simulink model "bd_inv_cont_3tank"  (R2021b)
settings: Solver=VariableStepAuto  StartTime=0.0  StopTime=1000  RelTol=1e-3
libraries: dspsrcs4 x4
settings Model: Creator=billtubbs  LastModifiedBy=billtubbs

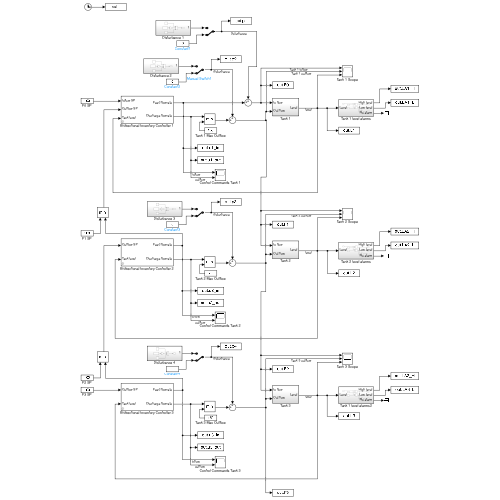
[thumbnail: Simulink's stored preview of the top-level diagram]
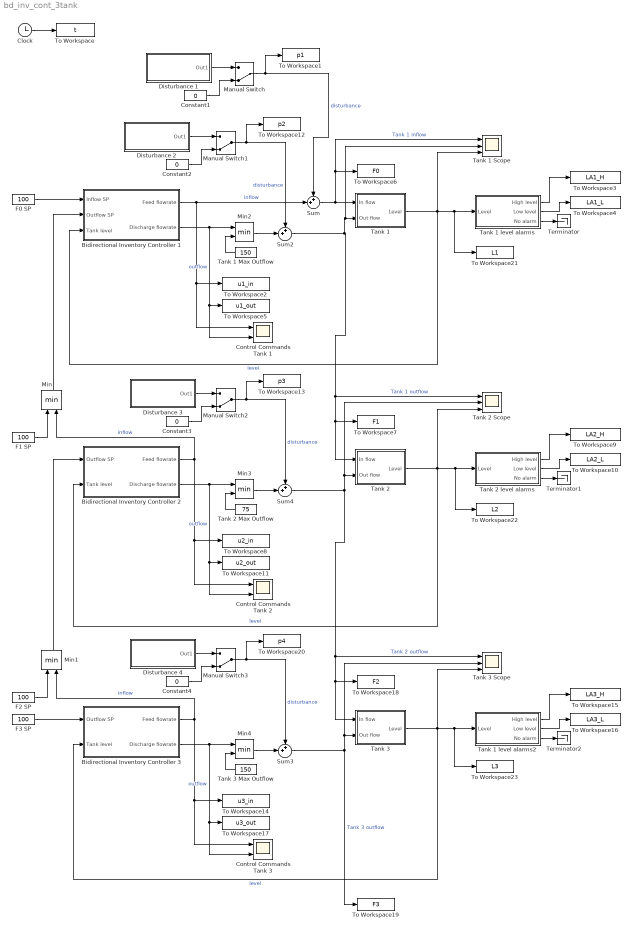
== system bd_inv_cont_3tank ==
  Bidirectional Inventory Controller 1 : Subsystem  mask{K=5, Ti=40, Tsp=40, u_nop=50}
  Bidirectional Inventory Controller 2 : Subsystem  mask{K=5, Ti=40, Tsp=40, u_nop=50}
  Bidirectional Inventory Controller 3 : Subsystem  mask{K=5, Ti=40, Tsp=40, u_nop=50}
  Clock : Clock
  Constant{1..4} (4 alike) : Constant  Value=0  SampleTime=1
  Control Commands Tank 1 : Scope  NumInputPorts=2
  Control Commands Tank 2 : Scope  NumInputPorts=2
  Control Commands Tank 3 : Scope  NumInputPorts=2
  Disturbance 1 : Subsystem
  Disturbance 2 : Subsystem
  Disturbance 3 : Subsystem
  Disturbance 4 : Subsystem
  F0 SP : Constant  Value=100
  F1 SP : Constant  Value=100  VectorParams1D=off
  F2 SP : Constant  Value=100
  F3 SP : Constant  Value=100  VectorParams1D=off
  Manual Switch{,1..3} (4 alike) : ManualSwitch  CurrentSetting=0
  Min{,1..4} (5 alike) : MinMax  Inputs=2
  Sum{,2..4} (4 alike) : Sum  Inputs=++|
  Tank 1 : Subsystem
  Tank 1 Max Outflow : Constant  Value=150
  Tank 1 Scope : Scope  NumInputPorts=3
  Tank 1 level alarms : Subsystem
  Tank 1 level alarms2 : Subsystem
  Tank 2 : Subsystem
  Tank 2 Max Outflow : Constant  Value=75
  Tank 2 Scope : Scope  NumInputPorts=3
  Tank 2 level alarms : Subsystem
  Tank 3 : Subsystem
  Tank 3 Max Outflow : Constant  Value=150
  Tank 3 Scope : Scope  NumInputPorts=3
  Terminator : Terminator
  Terminator1 : Terminator
  Terminator2 : Terminator
  To Workspace : ToWorkspace  VariableName=t  SampleTime=1
  To Workspace1 : ToWorkspace  VariableName=p1  SampleTime=1
      settings: Save2DSignal=2-D array (concatenate along first dimension)
  To Workspace10 : ToWorkspace  VariableName=LA2_L  SampleTime=1
  To Workspace11 : ToWorkspace  VariableName=u2_out  SampleTime=1
  To Workspace12 : ToWorkspace  VariableName=p2  SampleTime=1
      settings: Save2DSignal=2-D array (concatenate along first dimension)
  To Workspace13 : ToWorkspace  VariableName=p3  SampleTime=1
      settings: Save2DSignal=2-D array (concatenate along first dimension)
  To Workspace14 : ToWorkspace  VariableName=u3_in  SampleTime=1
  To Workspace15 : ToWorkspace  VariableName=LA3_H  SampleTime=1
  To Workspace16 : ToWorkspace  VariableName=LA3_L  SampleTime=1
  To Workspace17 : ToWorkspace  VariableName=u3_out  SampleTime=1
  To Workspace18 : ToWorkspace  VariableName=F2  SampleTime=1
  To Workspace19 : ToWorkspace  VariableName=F3  SampleTime=1
  To Workspace2 : ToWorkspace  VariableName=u1_in  SampleTime=1
  To Workspace20 : ToWorkspace  VariableName=p4  SampleTime=1
      settings: Save2DSignal=2-D array (concatenate along first dimension)
  To Workspace21 : ToWorkspace  VariableName=L1  SampleTime=1
  To Workspace22 : ToWorkspace  VariableName=L2  SampleTime=1
  To Workspace23 : ToWorkspace  VariableName=L3  SampleTime=1
  To Workspace3 : ToWorkspace  VariableName=LA1_H  SampleTime=1
  To Workspace4 : ToWorkspace  VariableName=LA1_L  SampleTime=1
  To Workspace5 : ToWorkspace  VariableName=u1_out  SampleTime=1
  To Workspace6 : ToWorkspace  VariableName=F0  SampleTime=1
  To Workspace7 : ToWorkspace  VariableName=F1  SampleTime=1
  To Workspace8 : ToWorkspace  VariableName=u2_in  SampleTime=1
  To Workspace9 : ToWorkspace  VariableName=LA2_H  SampleTime=1
  wires:
  Clock/1 -> To Workspace/1
  Bidirectional Inventory Controller 1/2(Discharge flowrate) -> Min2/1, Control Commands Tank 1/2, To Workspace5/1  "outflow"
  Tank 1 level alarms/3(No alarm) -> Terminator/1
  Sum/1 -> Tank 1/1(In flow), Tank 1 Scope/1, To Workspace6/1  "Tank 1 inflow"
  Manual Switch/1 -> Sum/1, To Workspace1/1  "disturbance"
  Tank 1 level alarms/1(High level) -> To Workspace3/1
  Tank 1 level alarms/2(Low level) -> To Workspace4/1
  Bidirectional Inventory Controller 1/1(Feed flowrate) -> To Workspace2/1, Control Commands Tank 1/1, Sum/2  "inflow"
  Tank 1/1(Level) -> Tank 1 Scope/3, Bidirectional Inventory Controller 1/3(Tank level), To Workspace21/1, Tank 1 level alarms/1(Level)  "level"
  Constant1/1 -> Manual Switch/2
  F0 SP/1 -> Bidirectional Inventory Controller 1/1(Inflow SP)
  F1 SP/1 -> Min/1
  Min1/1 -> Bidirectional Inventory Controller 2/1(Outflow SP)
  Bidirectional Inventory Controller 2/1(Feed flowrate) -> To Workspace8/1, Control Commands Tank 2/1, Min/2  "inflow"
  Tank 2 level alarms/1(High level) -> To Workspace9/1
  Tank 2/1(Level) -> Bidirectional Inventory Controller 2/2(Tank level), Tank 2 Scope/3, To Workspace22/1, Tank 2 level alarms/1(Level)  "level"
  Tank 2 level alarms/2(Low level) -> To Workspace10/1
  Tank 2 level alarms/3(No alarm) -> Terminator1/1
  Sum2/1 -> Tank 2 Scope/1, Tank 2/1(In flow), To Workspace7/1, Tank 1 Scope/2, Tank 1/2(Out flow)  "Tank 1 outflow"
  Bidirectional Inventory Controller 2/2(Discharge flowrate) -> Min3/1, Control Commands Tank 2/2, To Workspace11/1  "outflow"
  F3 SP/1 -> Bidirectional Inventory Controller 3/1(Outflow SP)
  Bidirectional Inventory Controller 3/1(Feed flowrate) -> To Workspace14/1, Control Commands Tank 3/1, Min1/2  "inflow"
  Tank 1 level alarms2/1(High level) -> To Workspace15/1
  Tank 3/1(Level) -> Bidirectional Inventory Controller 3/2(Tank level), Tank 3 Scope/3, To Workspace23/1, Tank 1 level alarms2/1(Level)  "level"
  Tank 1 level alarms2/2(Low level) -> To Workspace16/1
  Tank 1 level alarms2/3(No alarm) -> Terminator2/1
  Bidirectional Inventory Controller 3/2(Discharge flowrate) -> Min4/1, Control Commands Tank 3/2, To Workspace17/1  "outflow"
  Min/1 -> Bidirectional Inventory Controller 1/2(Outflow SP)
  F2 SP/1 -> Min1/1
  Tank 1 Max Outflow/1 -> Min2/2
  Min2/1 -> Sum2/2
  Tank 2 Max Outflow/1 -> Min3/2
  Min3/1 -> Sum4/2
  Sum4/1 -> Tank 3 Scope/1, Tank 3/1(In flow), To Workspace18/1, Tank 2 Scope/2, Tank 2/2(Out flow)  "Tank 2 outflow"
  Min4/1 -> Sum3/2
  Tank 3 Max Outflow/1 -> Min4/2
  Sum3/1 -> To Workspace19/1, Tank 3 Scope/2, Tank 3/2(Out flow)  "Tank 3 outflow"
  Disturbance 1/1(Out1) -> Manual Switch/1
  Constant2/1 -> Manual Switch1/2
  Manual Switch1/1 -> Sum2/1, To Workspace12/1  "disturbance"
  Constant3/1 -> Manual Switch2/2
  Manual Switch2/1 -> Sum4/1, To Workspace13/1  "disturbance"
  Disturbance 3/1(Out1) -> Manual Switch2/1
  Constant4/1 -> Manual Switch3/2
  Disturbance 4/1(Out1) -> Manual Switch3/1
  Manual Switch3/1 -> Sum3/1, To Workspace20/1  "disturbance"
  Disturbance 2/1(Out1) -> Manual Switch1/1

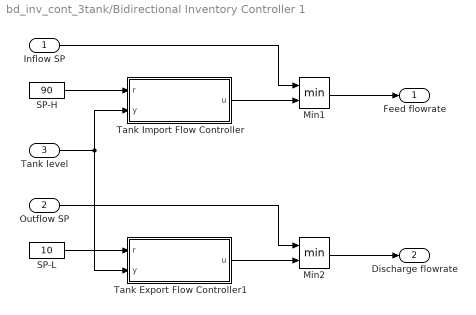
== system bd_inv_cont_3tank/Bidirectional Inventory Controller 1 ==
  Inflow SP : Inport
  Outflow SP : Inport  Port=2
  Tank level : Inport  Port=3
  Min1 : MinMax  Inputs=2
  Min2 : MinMax  Inputs=2
  SP-H : Constant  Value=90
  SP-L : Constant  Value=10
  Tank Export Flow Controller1 : Subsystem
  Tank Import Flow Controller : Subsystem
  Feed flowrate : Outport
  Discharge flowrate : Outport  Port=2
  wires:
  Tank Import Flow Controller/1(u) -> Min1/2
  Outflow SP/1 -> Min2/1
  Tank Export Flow Controller1/1(u) -> Min2/2
  Tank level/1 -> Tank Export Flow Controller1/2(y), Tank Import Flow Controller/2(y)
  SP-H/1 -> Tank Import Flow Controller/1(r)
  SP-L/1 -> Tank Export Flow Controller1/1(r)
  Inflow SP/1 -> Min1/1
  Min1/1 -> Feed flowrate/1
  Min2/1 -> Discharge flowrate/1

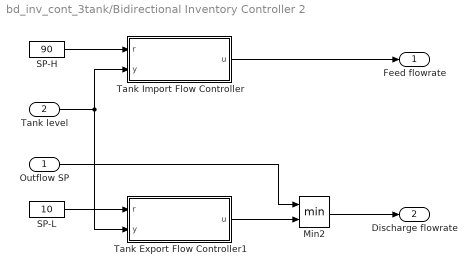
== system bd_inv_cont_3tank/Bidirectional Inventory Controller 2 ==
  Outflow SP : Inport
  Tank level : Inport  Port=2
  Min2 : MinMax  Inputs=2
  SP-H : Constant  Value=90
  SP-L : Constant  Value=10
  Tank Export Flow Controller1 : Subsystem
  Tank Import Flow Controller : Subsystem
  Feed flowrate : Outport
  Discharge flowrate : Outport  Port=2
  wires:
  Tank Import Flow Controller/1(u) -> Feed flowrate/1
  Outflow SP/1 -> Min2/1
  Tank Export Flow Controller1/1(u) -> Min2/2
  Tank level/1 -> Tank Export Flow Controller1/2(y), Tank Import Flow Controller/2(y)
  SP-H/1 -> Tank Import Flow Controller/1(r)
  SP-L/1 -> Tank Export Flow Controller1/1(r)
  Min2/1 -> Discharge flowrate/1

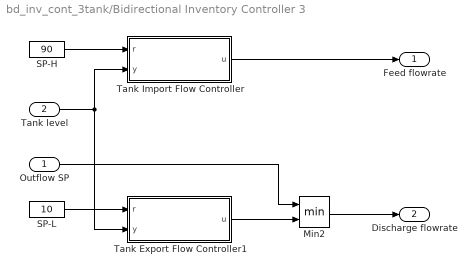
== system bd_inv_cont_3tank/Bidirectional Inventory Controller 3 ==
  Outflow SP : Inport
  Tank level : Inport  Port=2
  Min2 : MinMax  Inputs=2
  SP-H : Constant  Value=90
  SP-L : Constant  Value=10
  Tank Export Flow Controller1 : Subsystem
  Tank Import Flow Controller : Subsystem
  Feed flowrate : Outport
  Discharge flowrate : Outport  Port=2
  wires:
  Tank Import Flow Controller/1(u) -> Feed flowrate/1
  Outflow SP/1 -> Min2/1
  Tank Export Flow Controller1/1(u) -> Min2/2
  Tank level/1 -> Tank Export Flow Controller1/2(y), Tank Import Flow Controller/2(y)
  SP-H/1 -> Tank Import Flow Controller/1(r)
  SP-L/1 -> Tank Export Flow Controller1/1(r)
  Min2/1 -> Discharge flowrate/1

== system bd_inv_cont_3tank/Disturbance 1 ==
  Add : Sum  Inputs=+++
  Colored Noise : dspsrcs4/Colored Noise  Color=pink  InverseFrequencyPower=1  BoundedOutput=off  NumChannels=1  OutputDataType=double  SamplesPerFrame=1  SampleTime=1  RandomStream=mt19937ar with seed  Seed=67  SimulateUsing=Interpreted execution
      settings: SourceProductBaseCode=DS
  Gain : Gain  Gain=3
  Sine Wave : Sin  Amplitude=5  Frequency=1/60  SampleTime=0
  Step : Step  Time=100  After=0  SampleTime=0
  Out1 : Outport
  wires:
  Colored Noise/1 -> Gain/1
  Gain/1 -> Add/2
  Step/1 -> Add/3
  Sine Wave/1 -> Add/1
  Add/1 -> Out1/1

== system bd_inv_cont_3tank/Disturbance 2 ==
  Add : Sum  Inputs=+++
  Colored Noise : dspsrcs4/Colored Noise  Color=pink  InverseFrequencyPower=1  BoundedOutput=off  NumChannels=1  OutputDataType=double  SamplesPerFrame=1  SampleTime=1  RandomStream=mt19937ar with seed  Seed=67  SimulateUsing=Interpreted execution
      settings: SourceProductBaseCode=DS
  Gain : Gain  Gain=3
  Sine Wave : Sin  Amplitude=5  Frequency=1/60  SampleTime=0
  Step : Step  Time=100  After=0  SampleTime=0
  Out1 : Outport
  wires:
  Colored Noise/1 -> Gain/1
  Gain/1 -> Add/2
  Step/1 -> Add/3
  Sine Wave/1 -> Add/1
  Add/1 -> Out1/1

== system bd_inv_cont_3tank/Disturbance 3 ==
  Add : Sum  Inputs=+++
  Colored Noise : dspsrcs4/Colored Noise  Color=pink  InverseFrequencyPower=1  BoundedOutput=off  NumChannels=1  OutputDataType=double  SamplesPerFrame=1  SampleTime=1  RandomStream=mt19937ar with seed  Seed=67  SimulateUsing=Interpreted execution
      settings: SourceProductBaseCode=DS
  Gain : Gain  Gain=3
  Sine Wave : Sin  Amplitude=5  Frequency=1/60  SampleTime=0
  Step : Step  Time=100  After=0  SampleTime=0
  Out1 : Outport
  wires:
  Colored Noise/1 -> Gain/1
  Gain/1 -> Add/2
  Step/1 -> Add/3
  Sine Wave/1 -> Add/1
  Add/1 -> Out1/1

== system bd_inv_cont_3tank/Disturbance 4 ==
  Add : Sum  Inputs=+++
  Colored Noise : dspsrcs4/Colored Noise  Color=pink  InverseFrequencyPower=1  BoundedOutput=off  NumChannels=1  OutputDataType=double  SamplesPerFrame=1  SampleTime=1  RandomStream=mt19937ar with seed  Seed=67  SimulateUsing=Interpreted execution
      settings: SourceProductBaseCode=DS
  Gain : Gain  Gain=3
  Sine Wave : Sin  Amplitude=5  Frequency=1/60  SampleTime=0
  Step : Step  Time=100  After=0  SampleTime=0
  Out1 : Outport
  wires:
  Colored Noise/1 -> Gain/1
  Gain/1 -> Add/2
  Step/1 -> Add/3
  Sine Wave/1 -> Add/1
  Add/1 -> Out1/1

== system bd_inv_cont_3tank/Tank 1 ==
  In flow : Inport
  Out flow : Inport  Port=2
  Gain : Gain  Gain=0.05
  Integrator : Integrator
  Sum : Sum  Inputs=|+-
  Transport Delay : TransportDelay  Commented=on  DelayTime=0
  Level : Outport  InitialOutput=0
  wires:
  Sum/1 -> Gain/1
  Integrator/1 -> Level/1
  In flow/1 -> Sum/1
  Out flow/1 -> Sum/2
  Gain/1 -> Integrator/1

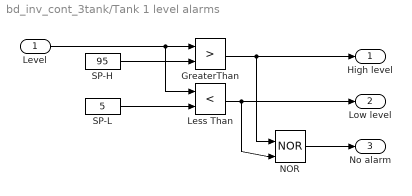
== system bd_inv_cont_3tank/Tank 1 level alarms ==
  Level : Inport
  GreaterThan : RelationalOperator  Operator=>  OutDataTypeStr=boolean  RndMeth=Simplest
  Less Than : RelationalOperator  Operator=<  OutDataTypeStr=boolean  RndMeth=Simplest
  NOR : Logic  Operator=NOR  IconShape=distinctive  AllPortsSameDT=off  OutDataTypeStr=boolean
  SP-H : Constant  Value=95
  SP-L : Constant  Value=5
  High level : Outport
  Low level : Outport  Port=2
  No alarm : Outport  Port=3
  wires:
  Level/1 -> Less Than/1, GreaterThan/1
  SP-L/1 -> Less Than/2
  GreaterThan/1 -> High level/1, NOR/1
  SP-H/1 -> GreaterThan/2
  Less Than/1 -> NOR/2, Low level/1
  NOR/1 -> No alarm/1

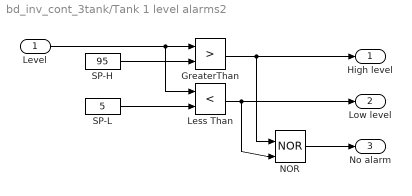
== system bd_inv_cont_3tank/Tank 1 level alarms2 ==
  Level : Inport
  GreaterThan : RelationalOperator  Operator=>  OutDataTypeStr=boolean  RndMeth=Simplest
  Less Than : RelationalOperator  Operator=<  OutDataTypeStr=boolean  RndMeth=Simplest
  NOR : Logic  Operator=NOR  IconShape=distinctive  AllPortsSameDT=off  OutDataTypeStr=boolean
  SP-H : Constant  Value=95
  SP-L : Constant  Value=5
  High level : Outport
  Low level : Outport  Port=2
  No alarm : Outport  Port=3
  wires:
  Level/1 -> Less Than/1, GreaterThan/1
  SP-L/1 -> Less Than/2
  GreaterThan/1 -> High level/1, NOR/1
  SP-H/1 -> GreaterThan/2
  Less Than/1 -> NOR/2, Low level/1
  NOR/1 -> No alarm/1

== system bd_inv_cont_3tank/Tank 2 ==
  In flow : Inport
  Out flow : Inport  Port=2
  Gain : Gain  Gain=0.05
  Integrator : Integrator
  Sum : Sum  Inputs=|+-
  Transport Delay : TransportDelay  Commented=on  DelayTime=0
  Level : Outport  InitialOutput=0
  wires:
  Sum/1 -> Gain/1
  Integrator/1 -> Level/1
  In flow/1 -> Sum/1
  Out flow/1 -> Sum/2
  Gain/1 -> Integrator/1

== system bd_inv_cont_3tank/Tank 2 level alarms ==
  Level : Inport
  GreaterThan : RelationalOperator  Operator=>  OutDataTypeStr=boolean  RndMeth=Simplest
  Less Than : RelationalOperator  Operator=<  OutDataTypeStr=boolean  RndMeth=Simplest
  NOR : Logic  Operator=NOR  IconShape=distinctive  AllPortsSameDT=off  OutDataTypeStr=boolean
  SP-H : Constant  Value=95
  SP-L : Constant  Value=5
  High level : Outport
  Low level : Outport  Port=2
  No alarm : Outport  Port=3
  wires:
  Level/1 -> Less Than/1, GreaterThan/1
  SP-L/1 -> Less Than/2
  GreaterThan/1 -> High level/1, NOR/1
  SP-H/1 -> GreaterThan/2
  Less Than/1 -> NOR/2, Low level/1
  NOR/1 -> No alarm/1

== system bd_inv_cont_3tank/Tank 3 ==
  In flow : Inport
  Out flow : Inport  Port=2
  Gain : Gain  Gain=0.05
  Integrator : Integrator
  Sum : Sum  Inputs=|+-
  Transport Delay : TransportDelay  Commented=on  DelayTime=0
  Level : Outport  InitialOutput=0
  wires:
  Sum/1 -> Gain/1
  Integrator/1 -> Level/1
  In flow/1 -> Sum/1
  Out flow/1 -> Sum/2
  Gain/1 -> Integrator/1

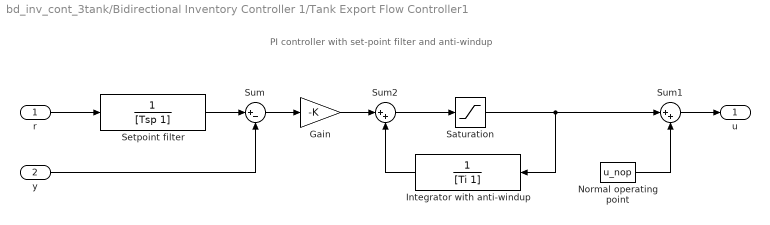
== system bd_inv_cont_3tank/Bidirectional Inventory Controller 1/Tank Export Flow Controller1 ==
  note: PI controller with set-point filter and anti-windup
  r : Inport
  y : Inport  Port=2
  Gain : Gain  Gain=-K
  Integrator with anti-windup : TransferFcn  Denominator=[Ti 1]
  Normal operating point : Constant  Value=u_nop
  Saturation : Saturate  UpperLimit=50  LowerLimit=-50
  Setpoint filter : TransferFcn  Denominator=[Tsp 1]
  Sum : Sum  Inputs=|+-
  Sum1 : Sum  Inputs=|++
  Sum2 : Sum  Inputs=|++
  u : Outport
  wires:
  r/1 -> Setpoint filter/1
  Sum1/1 -> u/1
  Saturation/1 -> Integrator with anti-windup/1, Sum1/1
  Normal operating point/1 -> Sum1/2
  Sum/1 -> Gain/1
  y/1 -> Sum/2
  Integrator with anti-windup/1 -> Sum2/2
  Sum2/1 -> Saturation/1
  Gain/1 -> Sum2/1
  Setpoint filter/1 -> Sum/1

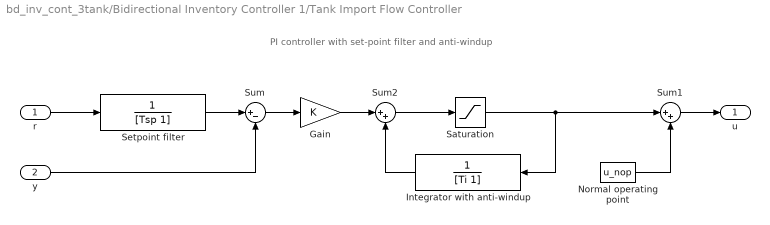
== system bd_inv_cont_3tank/Bidirectional Inventory Controller 1/Tank Import Flow Controller ==
  note: PI controller with set-point filter and anti-windup
  r : Inport
  y : Inport  Port=2
  Gain : Gain  Gain=K
  Integrator with anti-windup : TransferFcn  Denominator=[Ti 1]
  Normal operating point : Constant  Value=u_nop
  Saturation : Saturate  UpperLimit=50  LowerLimit=-50
  Setpoint filter : TransferFcn  Denominator=[Tsp 1]
  Sum : Sum  Inputs=|+-
  Sum1 : Sum  Inputs=|++
  Sum2 : Sum  Inputs=|++
  u : Outport
  wires:
  r/1 -> Setpoint filter/1
  Sum1/1 -> u/1
  Saturation/1 -> Integrator with anti-windup/1, Sum1/1
  Normal operating point/1 -> Sum1/2
  Sum/1 -> Gain/1
  y/1 -> Sum/2
  Integrator with anti-windup/1 -> Sum2/2
  Sum2/1 -> Saturation/1
  Gain/1 -> Sum2/1
  Setpoint filter/1 -> Sum/1

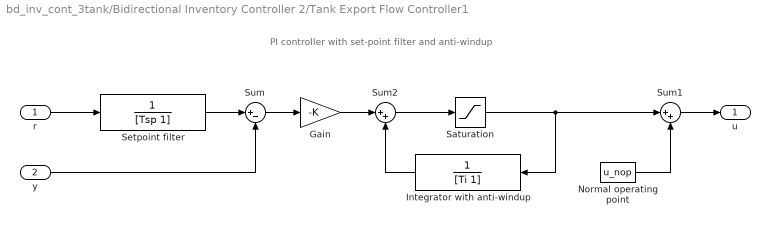
== system bd_inv_cont_3tank/Bidirectional Inventory Controller 2/Tank Export Flow Controller1 ==
  note: PI controller with set-point filter and anti-windup
  r : Inport
  y : Inport  Port=2
  Gain : Gain  Gain=-K
  Integrator with anti-windup : TransferFcn  Denominator=[Ti 1]
  Normal operating point : Constant  Value=u_nop
  Saturation : Saturate  UpperLimit=50  LowerLimit=-50
  Setpoint filter : TransferFcn  Denominator=[Tsp 1]
  Sum : Sum  Inputs=|+-
  Sum1 : Sum  Inputs=|++
  Sum2 : Sum  Inputs=|++
  u : Outport
  wires:
  r/1 -> Setpoint filter/1
  Sum1/1 -> u/1
  Saturation/1 -> Integrator with anti-windup/1, Sum1/1
  Normal operating point/1 -> Sum1/2
  Sum/1 -> Gain/1
  y/1 -> Sum/2
  Integrator with anti-windup/1 -> Sum2/2
  Sum2/1 -> Saturation/1
  Gain/1 -> Sum2/1
  Setpoint filter/1 -> Sum/1

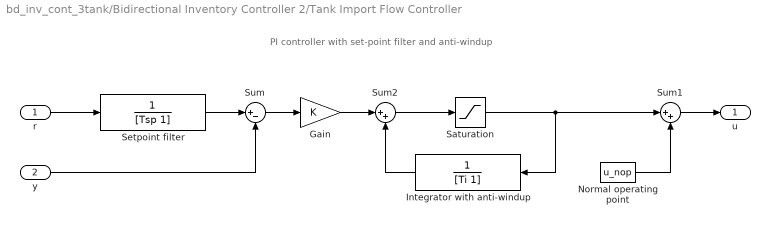
== system bd_inv_cont_3tank/Bidirectional Inventory Controller 2/Tank Import Flow Controller ==
  note: PI controller with set-point filter and anti-windup
  r : Inport
  y : Inport  Port=2
  Gain : Gain  Gain=K
  Integrator with anti-windup : TransferFcn  Denominator=[Ti 1]
  Normal operating point : Constant  Value=u_nop
  Saturation : Saturate  UpperLimit=50  LowerLimit=-50
  Setpoint filter : TransferFcn  Denominator=[Tsp 1]
  Sum : Sum  Inputs=|+-
  Sum1 : Sum  Inputs=|++
  Sum2 : Sum  Inputs=|++
  u : Outport
  wires:
  r/1 -> Setpoint filter/1
  Sum1/1 -> u/1
  Saturation/1 -> Integrator with anti-windup/1, Sum1/1
  Normal operating point/1 -> Sum1/2
  Sum/1 -> Gain/1
  y/1 -> Sum/2
  Integrator with anti-windup/1 -> Sum2/2
  Sum2/1 -> Saturation/1
  Gain/1 -> Sum2/1
  Setpoint filter/1 -> Sum/1

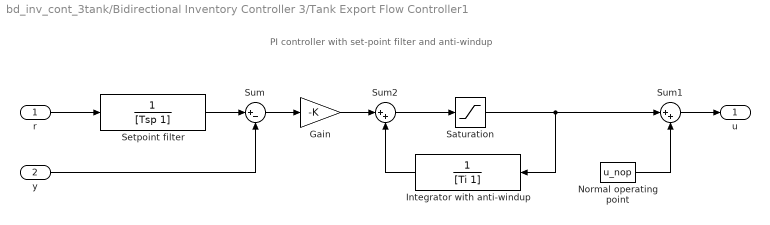
== system bd_inv_cont_3tank/Bidirectional Inventory Controller 3/Tank Export Flow Controller1 ==
  note: PI controller with set-point filter and anti-windup
  r : Inport
  y : Inport  Port=2
  Gain : Gain  Gain=-K
  Integrator with anti-windup : TransferFcn  Denominator=[Ti 1]
  Normal operating point : Constant  Value=u_nop
  Saturation : Saturate  UpperLimit=50  LowerLimit=-50
  Setpoint filter : TransferFcn  Denominator=[Tsp 1]
  Sum : Sum  Inputs=|+-
  Sum1 : Sum  Inputs=|++
  Sum2 : Sum  Inputs=|++
  u : Outport
  wires:
  r/1 -> Setpoint filter/1
  Sum1/1 -> u/1
  Saturation/1 -> Integrator with anti-windup/1, Sum1/1
  Normal operating point/1 -> Sum1/2
  Sum/1 -> Gain/1
  y/1 -> Sum/2
  Integrator with anti-windup/1 -> Sum2/2
  Sum2/1 -> Saturation/1
  Gain/1 -> Sum2/1
  Setpoint filter/1 -> Sum/1

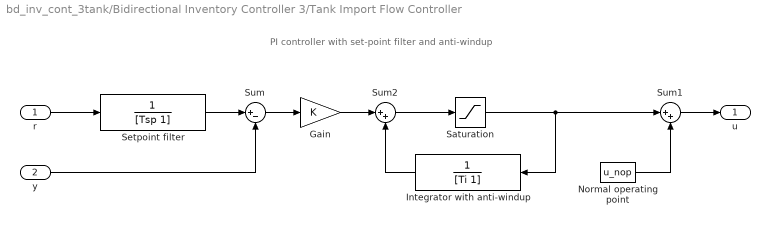
== system bd_inv_cont_3tank/Bidirectional Inventory Controller 3/Tank Import Flow Controller ==
  note: PI controller with set-point filter and anti-windup
  r : Inport
  y : Inport  Port=2
  Gain : Gain  Gain=K
  Integrator with anti-windup : TransferFcn  Denominator=[Ti 1]
  Normal operating point : Constant  Value=u_nop
  Saturation : Saturate  UpperLimit=50  LowerLimit=-50
  Setpoint filter : TransferFcn  Denominator=[Tsp 1]
  Sum : Sum  Inputs=|+-
  Sum1 : Sum  Inputs=|++
  Sum2 : Sum  Inputs=|++
  u : Outport
  wires:
  r/1 -> Setpoint filter/1
  Sum1/1 -> u/1
  Saturation/1 -> Integrator with anti-windup/1, Sum1/1
  Normal operating point/1 -> Sum1/2
  Sum/1 -> Gain/1
  y/1 -> Sum/2
  Integrator with anti-windup/1 -> Sum2/2
  Sum2/1 -> Saturation/1
  Gain/1 -> Sum2/1
  Setpoint filter/1 -> Sum/1
